simulink model "nadrz_fuzzy_1c"  (R2023a)
settings: Solver=ode45  StartTime=0.0  StopTime=200  FixedStep=0.01  MaxStep=0.2  RelTol=1e-3  EnableMultiTasking=on
libraries: fuzblock x2
settings Model: Creator=Ivan  LastModifiedBy=laptop
settings SolverCC: AlgebraicLoopSolver=TrustRegion
settings DataIOCC: LimitDataPoints=on  SaveFormat=Array  SignalLoggingSaveFormat=ModelDataLogs  ReturnWorkspaceOutputs=off  SignalLoggingName=sigsOut
settings OptimizationCC: BooleanDataType=off  InitFltsAndDblsToZero=on  LifeSpan=inf
settings DebuggingCC: SaveWithParameterizedLinksMsg=none  UnderspecifiedInitializationDetection=Classic  MergeDetectMultiDrivingBlocksExec=none  SignalResolutionControl=TryResolveAllWithWarning  MultiTaskDSMMsg=warning  MultiTaskCondExecSysMsg=none  FcnCallInpInsideContextMsg=warning  UnconnectedInputMsg=warning  UnconnectedOutputMsg=warning  UnconnectedLineMsg=warning  SFUnexpectedBacktrackingDiag=warning  SFNoUnconditionalDefaultTransitionDiag=warning  SFExecutionAtInitializationDiag=none  ArithmeticOperatorsInVariantConditions=warning
settings HardwareCC: ProdBitPerPointer=32  ProdBitPerSizeT=32  ProdBitPerPtrDiffT=32  ProdLargestAtomicFloat=None  ProdIntDivRoundTo=Undefined  ProdEndianess=Unspecified  ProdWordSize=32  ProdHWDeviceType=32-bit Generic  TargetUnknown=on
settings ModelReferenceCC: EnableRefExpFcnMdlSchedulingChecks=on  PropagateSignalLabelsOutOfModel=off
settings SFSimCC: SimUseLocalCustomCode=off  CustomCodeUndefinedFunction=UseInterfaceOnly
settings RTWCC: RTWUseLocalCustomCode=off  DLArmComputeVersion=19.05
settings CodeAppCC: StateflowObjectComments=on
settings GRTTargetCC: TargetFcnLib=ansi_tfl_tmw.mat  TargetLangStandard=C89/C90 (ANSI)  ModelReferenceCompliant=off  CombineOutputUpdateFcns=off  MatFileLogging=off  GRTInterface=on
settings ConfigComp: CovMetricSettings=dw  CovSaveCumulativeToWorkspaceVar=on  CovSaveSingleToWorkspaceVar=on  CovExternalEMLEnable=off

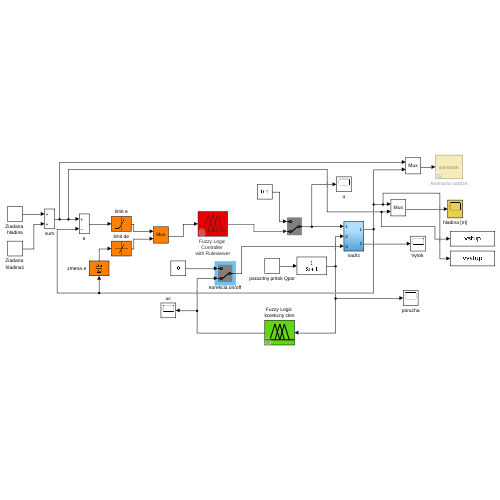
[thumbnail: Simulink's stored preview of the top-level diagram]
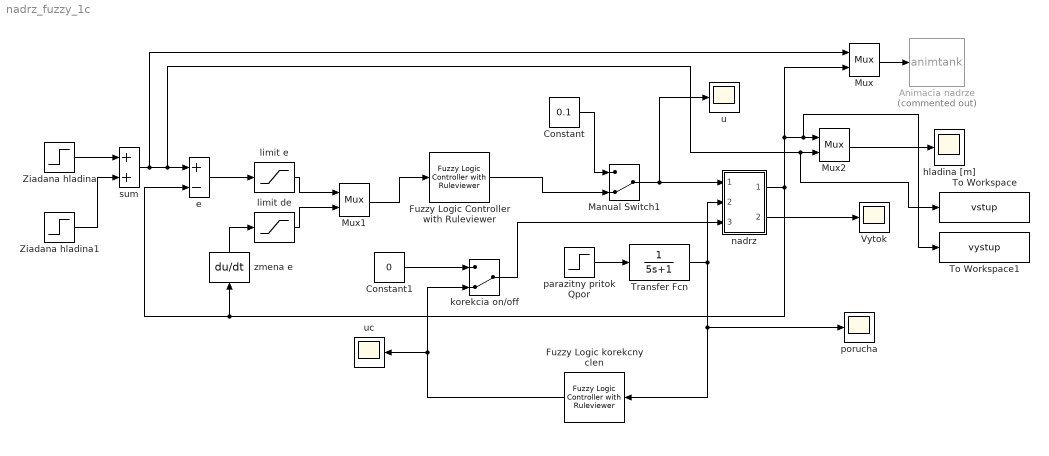
== system nadrz_fuzzy_1c ==
  Animacia nadrze : S-Function  Commented=on  FunctionName=animtank  Parameters=1  SFunctionDeploymentMode=off  EnableBusSupport=off
  Constant : Constant  Value=0.1
  Constant1 : Constant  Value=0
  Fuzzy Logic Controller with Ruleviewer : fuzblock/Fuzzy Logic  Controller  with Ruleviewer  fismatrix=fuzreg1  Ts=2
  Fuzzy Logic korekcny clen : fuzblock/Fuzzy Logic  Controller  with Ruleviewer  fismatrix=fuzkor1  Ts=2
  Manual Switch1 : ManualSwitch  CurrentSetting=0
  Mux : Mux  Inputs=2
  Mux1 : Mux  Inputs=2
  Mux2 : Mux  Inputs=2
  To Workspace : ToWorkspace  VariableName=vstup  SaveFormat=Timeseries  SampleTime=-1
  To Workspace1 : ToWorkspace  VariableName=vystup  SaveFormat=Timeseries  SampleTime=-1
  Transfer Fcn : TransferFcn  Denominator=[5 1]
  "Vytok " : Scope
  Ziadana hladina : Step  Time=5  After=1.5  SampleTime=0
  Ziadana hladina1 : Step  Time=60  After=-0.5  SampleTime=0
  e : Sum  Inputs=+-  InputSameDT=on  SaturateOnIntegerOverflow=on  OutDataTypeStr=Inherit: Same as first input
  hladina [m] : Scope
  korekcia on/off : ManualSwitch  CurrentSetting=0
  limit de : Saturate  UpperLimit=0.3  LowerLimit=-0.3
  limit e : Saturate  UpperLimit=2  LowerLimit=-2
  nadrz : Subsystem
  parazitny pritok Qpor : Step  Time=120  After=0.12  SampleTime=0
  porucha : Scope
  sum : Sum  InputSameDT=on  SaturateOnIntegerOverflow=on  OutDataTypeStr=Inherit: Same as first input
  u : Scope
  uc : Scope
  zmena e : Derivative
  wires:
  Mux/1 -> Animacia nadrze/1
  nadrz/1(Out1) -> To Workspace1/1, Mux2/1, Mux/2, zmena e/1, e/2
  Manual Switch1/1 -> nadrz/1(In1), u/1
  e/1 -> limit e/1
  nadrz/2(Out2) -> "Vytok "/1
  Constant/1 -> Manual Switch1/1
  Ziadana hladina/1 -> sum/1
  zmena e/1 -> limit de/1
  limit de/1 -> Mux1/2
  limit e/1 -> Mux1/1
  Mux1/1 -> Fuzzy Logic Controller with Ruleviewer/1
  Ziadana hladina1/1 -> sum/2
  Constant1/1 -> korekcia on/off/1
  Fuzzy Logic korekcny clen/1 -> korekcia on/off/2, uc/1
  Fuzzy Logic Controller with Ruleviewer/1 -> Manual Switch1/2
  parazitny pritok Qpor/1 -> Transfer Fcn/1
  Transfer Fcn/1 -> porucha/1, Fuzzy Logic korekcny clen/1, nadrz/2(In2)
  korekcia on/off/1 -> nadrz/3(In3)
  Mux2/1 -> hladina [m]/1
  sum/1 -> To Workspace/1, Mux2/2, e/1, Mux/1

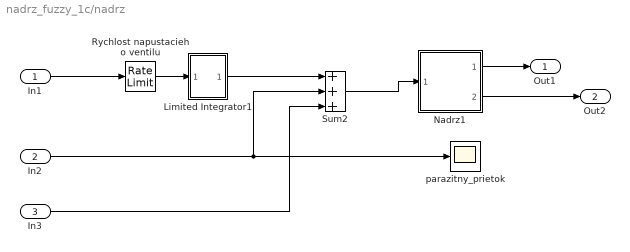
== system nadrz_fuzzy_1c/nadrz ==
  In1 : Inport
  In2 : Inport  Port=2
  In3 : Inport  Port=3
  Limited Integrator1 : Subsystem  mask(Limited integrator.){lb=0, ub=0.3, xi=0}
      mask prompts: lb "Lower bound:"; ub "Upper bound:"; xi "Initial condition"
      mask help: Limited integrator
      mask Help: Implements a limited integrator with \nan expression of the form:\n\nif(x<=lb and u<0) or (x>=ub and u>0)\n\txdot=0\nelse\n\txdot=u.
      mask Display: plot(-1,-0.2,3.5,1.2,[0.05,1,2,2.9],[0,0,1,1]);disp(' 1/s    ')
  Nadrz1 : Subsystem  mask(Water tank){ht=2, area=1, outletArea=0.05, overflowLimit=0, initialHt=0}
      mask prompts: ht "Height of tank (m):"; area "Bottom area (m^2):"; outletArea "Out pipe crossection (m^2):"; overflowLimit "Overflow sensor distance from top (m):"; initialHt "Initial level height (m):"
      mask help: Cylindrical water tank with overflow signal
      mask Display: disp('WATER\nTANK')
  Rychlost napustacieho ventilu : RateLimiter  RisingSlewLimit=0.015  FallingSlewLimit=-0.015
  Sum2 : Sum  Inputs=+++  InputSameDT=on  SaturateOnIntegerOverflow=on  OutDataTypeStr=Inherit: Same as first input
  parazitny_prietok : Scope
  Out1 : Outport
  Out2 : Outport  Port=2
  wires:
  Nadrz1/1(water level) -> Out1/1
  Nadrz1/2(flow out) -> Out2/1
  Rychlost napustacieho ventilu/1 -> Limited Integrator1/1(In_1)
  In1/1 -> Rychlost napustacieho ventilu/1
  In2/1 -> Sum2/2, parazitny_prietok/1
  Sum2/1 -> Nadrz1/1(flow in)
  Limited Integrator1/1(Out_1) -> Sum2/1
  In3/1 -> Sum2/3

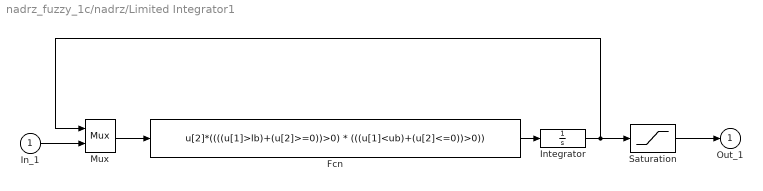
== system nadrz_fuzzy_1c/nadrz/Limited Integrator1 ==
  In_1 : Inport
  Fcn : Fcn  Expr=u[2]*((((u[1]>lb)+(u[2]>=0))>0) * (((u[1]<ub)+(u[2]<=0))>0))
  Integrator : Integrator  InitialCondition=xi
  Mux : Mux  Inputs=2
  Saturation : Saturate  UpperLimit=ub  LowerLimit=lb
  Out_1 : Outport  InitialOutput=0
  wires:
  Integrator/1 -> Saturation/1, Mux/1
  Fcn/1 -> Integrator/1
  Mux/1 -> Fcn/1
  In_1/1 -> Mux/2
  Saturation/1 -> Out_1/1

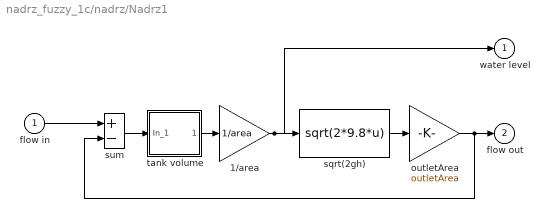
== system nadrz_fuzzy_1c/nadrz/Nadrz1 ==
  flow in : Inport
  1/area : Gain  Gain=1/area  SaturateOnIntegerOverflow=on  OutDataTypeStr=Inherit: Same as input  ParamDataTypeStr=Inherit: Same as input
  outletArea : Gain  Gain=outletArea  SaturateOnIntegerOverflow=on  OutDataTypeStr=Inherit: Same as input  ParamDataTypeStr=Inherit: Same as input
  sqrt(2gh) : Fcn  Expr=sqrt(2*9.8*u)
  sum : Sum  Inputs=+-  InputSameDT=on  SaturateOnIntegerOverflow=on  OutDataTypeStr=Inherit: Same as first input
  tank volume : Subsystem  mask(Limited integrator.){lb=0, ub=ht * area, xi=0}
      mask prompts: lb "Lower bound:"; ub "Upper bound:"; xi "Initial condition"
      mask help: Limited integrator
      mask Help: Implements a limited integrator with \nan expression of the form:\n\nif(x<=lb and u<0) or (x>=ub and u>0)\n\txdot=0\nelse\n\txdot=u.
      mask Display: plot(-1,-0.2,3.5,1.2,[0.05,1,2,2.9],[0,0,1,1]);disp(' 1/s    ')
  water level : Outport  InitialOutput=0
  flow out : Outport  Port=2  InitialOutput=0
  wires:
  outletArea/1 -> flow out/1, sum/2
  sqrt(2gh)/1 -> outletArea/1
  1/area/1 -> water level/1, sqrt(2gh)/1
  tank volume/1(Out_1) -> 1/area/1
  flow in/1 -> sum/1
  sum/1 -> tank volume/1(In_1)

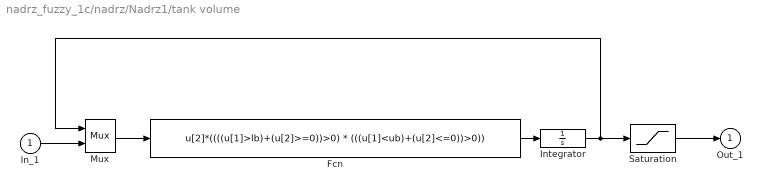
== system nadrz_fuzzy_1c/nadrz/Nadrz1/tank volume ==
  In_1 : Inport
  Fcn : Fcn  Expr=u[2]*((((u[1]>lb)+(u[2]>=0))>0) * (((u[1]<ub)+(u[2]<=0))>0))
  Integrator : Integrator  InitialCondition=xi
  Mux : Mux  Inputs=2
  Saturation : Saturate  UpperLimit=ub  LowerLimit=lb
  Out_1 : Outport  InitialOutput=0
  wires:
  Integrator/1 -> Saturation/1, Mux/1
  Fcn/1 -> Integrator/1
  Mux/1 -> Fcn/1
  In_1/1 -> Mux/2
  Saturation/1 -> Out_1/1
